simulink model "Ejercicio6v2_27_03_17"  (R2013a)
settings: Solver=ode23tb  StartTime=0.0  StopTime=1  RelTol=1e-3
libraries: powerlib x25
settings Model: Creator=Miguel  LastModifiedBy=Miguel

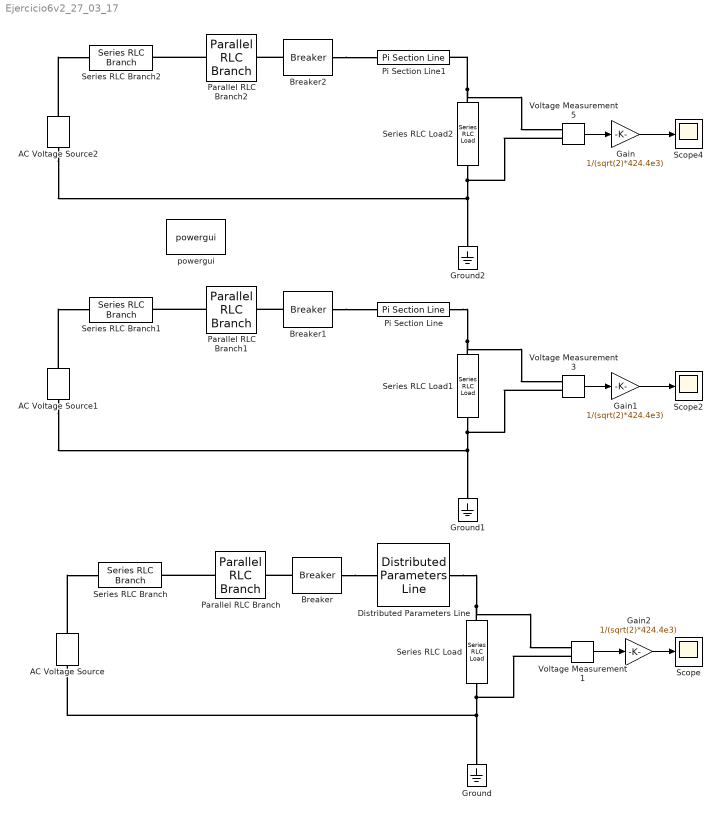
== system Ejercicio6v2_27_03_17 ==
  AC Voltage Source : powerlib/Electrical Sources/AC Voltage Source  Amplitude=sqrt(2)*424.4e3  Phase=0  Frequency=60  SampleTime=0  Measurements=None
  AC Voltage Source1 : powerlib/Electrical Sources/AC Voltage Source  Amplitude=sqrt(2)*424.4e3  Phase=0  Frequency=60  SampleTime=0  Measurements=None
  AC Voltage Source2 : powerlib/Electrical Sources/AC Voltage Source  Amplitude=sqrt(2)*424.4e3  Phase=0  Frequency=60  SampleTime=0  Measurements=None
  Breaker : powerlib/Elements/Breaker  BreakerResistance=0.001  InitialState=0  SnubberResistance=inf  SnubberCapacitance=0  SwitchingTimes=[(1/60)/4]  External=off  Measurements=None  MoreParameters=off  NoBreakLoop=off
  Breaker1 : powerlib/Elements/Breaker  BreakerResistance=0.001  InitialState=0  SnubberResistance=inf  SnubberCapacitance=0  SwitchingTimes=[(1/60)/4]  External=off  Measurements=None  MoreParameters=off  NoBreakLoop=off
  Breaker2 : powerlib/Elements/Breaker  BreakerResistance=0.001  InitialState=0  SnubberResistance=inf  SnubberCapacitance=0  SwitchingTimes=[(1/60)/4]  External=off  Measurements=None  MoreParameters=off  NoBreakLoop=off
  Distributed Parameters Line : powerlib/Elements/Distributed Parameters Line  Phases=1  Frequency=60  Resistance=[0.011]  Inductance=[0.8674e-3]  Capacitance=[13.41e-9]  Length=300  x1=[0 0;0.000204632847803084 0;0.000409265695606167 0;0.000613898543409251 0;0.000818531391212335 0;0.00102316423901542 0]  x2=[0 0;0.000204632847803084 0;0.000409265695606167 0;0.000613898543409251 0;0.000818531391212335 0;0.00102316423901542 0]  x3=[0 0;0.000204632847803084 0;0.000409265695606167 0;0.000613898543409251 0;0.000818531391212335 0;0.00102316423901542 0]  x4=[0 0;0.000204632847803084 0;0.000409265695606167 0;0.000613898543409251 0;0.000818531391212335 0;0.00102316423901542 0]  x5=0.00102316423901542  Measurements=None
  Gain : Gain  Gain=1/(sqrt(2)*424.4e3)
  Gain1 : Gain  Gain=1/(sqrt(2)*424.4e3)
  Gain2 : Gain  Gain=1/(sqrt(2)*424.4e3)
  Ground : powerlib/Elements/Ground  LConnTagsString=a
  Ground1 : powerlib/Elements/Ground  LConnTagsString=a
  Ground2 : powerlib/Elements/Ground  LConnTagsString=a
  Parallel RLC Branch : powerlib/Elements/Parallel RLC Branch  LConnTagsString=a  RConnTagsString=__new0  BranchType=RLC  Resistance=180.1  Inductance=26.525e-3  SetiL0=off  InitialCurrent=0  Capacitance=117.84e-6  Setx0=off  InitialVoltage=0  Measurements=None
  Parallel RLC Branch1 : powerlib/Elements/Parallel RLC Branch  LConnTagsString=a  RConnTagsString=__new0  BranchType=RLC  Resistance=180.1  Inductance=26.525e-3  SetiL0=off  InitialCurrent=0  Capacitance=117.84e-6  Setx0=off  InitialVoltage=0  Measurements=None
  Parallel RLC Branch2 : powerlib/Elements/Parallel RLC Branch  LConnTagsString=a  RConnTagsString=__new0  BranchType=RLC  Resistance=180.1  Inductance=26.525e-3  SetiL0=off  InitialCurrent=0  Capacitance=117.84e-6  Setx0=off  InitialVoltage=0  Measurements=None
  Pi Section Line : powerlib/Elements/Pi Section Line  LConnTagsString=__new0  RConnTagsString=__new0  Frequency=60  Resistance=0.011  Inductance=0.8674e-3  Capacitance=13.41e-9  Length=300  PiSections=10  Measurements=None
      settings: AttributesFormatString=\n
  Pi Section Line1 : powerlib/Elements/Pi Section Line  LConnTagsString=__new0  RConnTagsString=__new0  Frequency=60  Resistance=0.011  Inductance=0.8674e-3  Capacitance=13.41e-9  Length=300  PiSections=1  Measurements=Input and output voltages
      settings: AttributesFormatString=\n
  Scope : Scope
      settings: ShowLegends=on  SaveName=u2_3
  Scope2 : Scope
      settings: ShowLegends=on  SaveName=u2_2
  Scope4 : Scope
      settings: ShowLegends=on  SaveName=u2_1
  Series RLC Branch : powerlib/Elements/Series RLC Branch  LConnTagsString=__new0  RConnTagsString=__new0  BranchType=R  Resistance=2  Inductance=1e-3  SetiL0=off  InitialCurrent=0  Capacitance=1e-6  Setx0=off  InitialVoltage=0  Measurements=None
  Series RLC Branch1 : powerlib/Elements/Series RLC Branch  LConnTagsString=__new0  RConnTagsString=__new0  BranchType=R  Resistance=2  Inductance=1e-3  SetiL0=off  InitialCurrent=0  Capacitance=1e-6  Setx0=off  InitialVoltage=0  Measurements=None
  Series RLC Branch2 : powerlib/Elements/Series RLC Branch  LConnTagsString=__new0  RConnTagsString=__new0  BranchType=R  Resistance=2  Inductance=1e-3  SetiL0=off  InitialCurrent=0  Capacitance=1e-6  Setx0=off  InitialVoltage=0  Measurements=None
  Series RLC Load : powerlib/Elements/Series RLC Load  LConnTagsString=a  RConnTagsString=__new0  NominalVoltage=424.4e3  NominalFrequency=60  ActivePower=110e6/300  InductivePower=110e6  CapacitivePower=0  Setx0=off  InitialVoltage=0  SetiL0=off  InitialCurrent=0  Measurements=None
  Series RLC Load1 : powerlib/Elements/Series RLC Load  LConnTagsString=a  RConnTagsString=__new0  NominalVoltage=424.4e3  NominalFrequency=60  ActivePower=110e6/300  InductivePower=110e6  CapacitivePower=0  Setx0=off  InitialVoltage=0  SetiL0=off  InitialCurrent=0  Measurements=None
  Series RLC Load2 : powerlib/Elements/Series RLC Load  LConnTagsString=a  RConnTagsString=__new0  NominalVoltage=424.4e3  NominalFrequency=60  ActivePower=110e6/300  InductivePower=110e6  CapacitivePower=0  Setx0=off  InitialVoltage=0  SetiL0=off  InitialCurrent=0  Measurements=None
  Voltage Measurement1 : powerlib/Measurements/Voltage Measurement  PhasorSimulation=off  OutputType=Complex  PSBequivalent=0
  Voltage Measurement3 : powerlib/Measurements/Voltage Measurement  PhasorSimulation=off  OutputType=Complex  PSBequivalent=0
  Voltage Measurement5 : powerlib/Measurements/Voltage Measurement  PhasorSimulation=off  OutputType=Complex  PSBequivalent=0
  powergui : powerlib/powergui  Priority=1  SimulationMode=Continuous  SolverType=Tustin  SampleTime=50e-6  frequency=60  SPID=off  DisableSnubberDevices=off  DisableRonSwitches=off  DisableVfSwitches=off  SwTol=0  Interpol=off  DisplayEquations=off  frequencyindice=60  Pbase=100e6  ErrMax=1e-4  Iterations=50  UnitsV=kV  UnitsW=MW  FunctionMessages=off  echomessages=off  HookPort=off  EnableUseOfTLC=off  x0status=blocks  RestoreLinks=warning  ResistiveCurrentMeasurement=off  Frange=[0:2:500]  Ylog=off  Xlog=on  ShowGrid=off  save=off  variable=ZData  ZoomFFT=off  StartTime=0.0  cycles=1  DisplayStyle=1  fundamental=60  FreqAxis=off  MaxFrequency=1000  frequencyindicesteady=1  RmsSteady=1  display=off  Ts=0  methode=off
  wires:
  Voltage Measurement1/1 -> Gain2/1
  Voltage Measurement3/1 -> Gain1/1
  Voltage Measurement5/1 -> Gain/1
  Gain2/1 -> Scope/1
  Gain1/1 -> Scope2/1
  Gain/1 -> Scope4/1
  connections:
  Series RLC Load/LConn1 -- Voltage Measurement1/LConn1 -- Distributed Parameters Line/RConn1
  AC Voltage Source/LConn1 -- Ground/LConn1 -- Voltage Measurement1/LConn2 -- Series RLC Load/RConn1
  Breaker/RConn1 -- Distributed Parameters Line/LConn1
  AC Voltage Source/RConn1 -- Series RLC Branch/LConn1
  Parallel RLC Branch/LConn1 -- Series RLC Branch/RConn1
  Breaker/LConn1 -- Parallel RLC Branch/RConn1
  Series RLC Load1/LConn1 -- Voltage Measurement3/LConn1 -- Pi Section Line/RConn1
  AC Voltage Source1/LConn1 -- Ground1/LConn1 -- Voltage Measurement3/LConn2 -- Series RLC Load1/RConn1
  Breaker1/RConn1 -- Pi Section Line/LConn1
  Parallel RLC Branch1/LConn1 -- Series RLC Branch1/RConn1
  AC Voltage Source1/RConn1 -- Series RLC Branch1/LConn1
  Breaker1/LConn1 -- Parallel RLC Branch1/RConn1
  Series RLC Load2/LConn1 -- Pi Section Line1/RConn1 -- Voltage Measurement5/LConn1
  Series RLC Load2/RConn1 -- Voltage Measurement5/LConn2 -- Ground2/LConn1 -- AC Voltage Source2/LConn1
  Breaker2/RConn1 -- Pi Section Line1/LConn1
  Parallel RLC Branch2/LConn1 -- Series RLC Branch2/RConn1
  Breaker2/LConn1 -- Parallel RLC Branch2/RConn1
  AC Voltage Source2/RConn1 -- Series RLC Branch2/LConn1
